simulink model "U27Estim"  (R2022b)
settings: Solver=ode23  StartTime=0.0  StopTime=2  RelTol=1e-3
undefined symbols (not defined in the file or in its folder): b, f, J, Kcj, Lm, Lr, Ls, p, Rr, Rs, Vs
libraries: cstblocks x2, spsAsynchronousMachineSIUnitsLib x1, spsGroundLib x1, spsThreePhaseProgrammableVoltageSourceLib x1, spsThreePhaseVIMeasurementLib x1, spspowerguiLib x1, spsPLL3phLib x1, spsabctodq0Lib x1
settings Model: Creator=automatizacion  LastModifiedBy=electronica

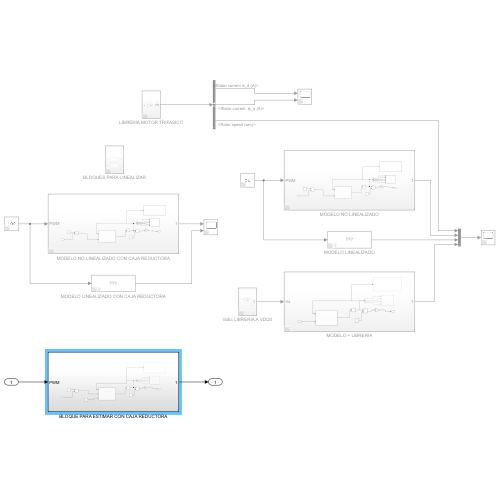
[thumbnail: Simulink's stored preview of the top-level diagram]
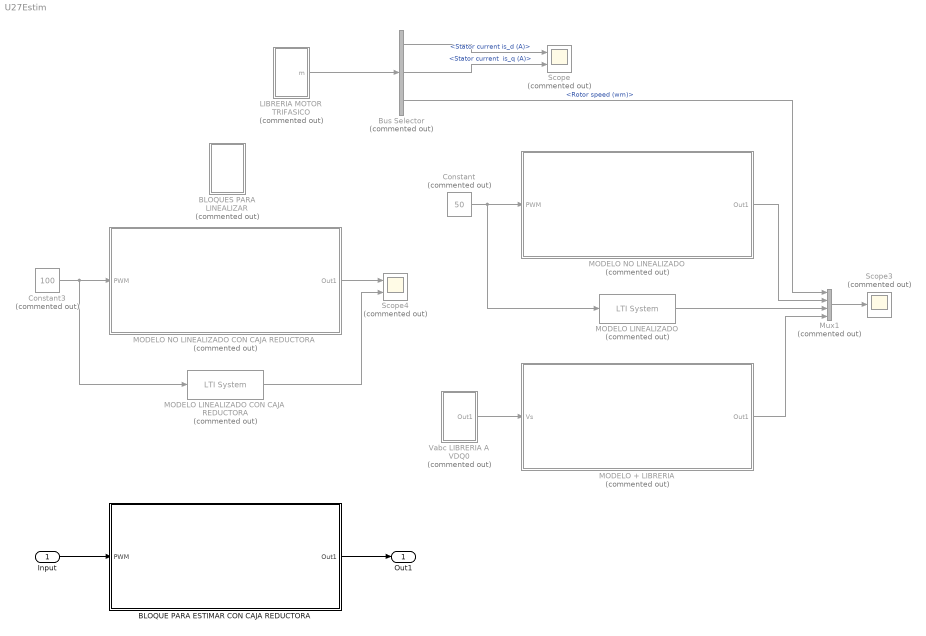
== system U27Estim ==
  Input : Inport
  BLOQUE PARA ESTIMAR CON CAJA REDUCTORA : Subsystem
  BLOQUES PARA LINEALIZAR : Subsystem  Commented=on
  Bus Selector : BusSelector  Commented=on  OutputSignals="Stator measurements.Stator current is_d (A),Stator measurements.Stator current  is_q (A),Mechanical.Rotor speed (wm)"
  Constant : Constant  Commented=on  Value=50
  Constant3 : Constant  Commented=on  Value=100
  LIBRERIA MOTOR TRIFASICO : Subsystem  Commented=on
  MODELO + LIBRERIA : Subsystem  Commented=on
  "MODELO LINEALIZADO " : cstblocks/LTI System  Commented=on  sys=G1  IC=[]
  MODELO LINEALIZADO CON CAJA REDUCTORA : cstblocks/LTI System  Commented=on  sys=G2  IC=[]
  "MODELO NO LINEALIZADO " : Subsystem  Commented=on
  MODELO NO LINEALIZADO CON CAJA REDUCTORA : Subsystem  Commented=on
  Mux1 : Mux  Commented=on
  Scope : Scope  Commented=on  NumInputPorts=2
  Scope3 : Scope  Commented=on
  Scope4 : Scope  Commented=on  NumInputPorts=2
  Vabc LIBRERIA A VDQ0 : Subsystem  Commented=on
  Out1 : Outport
  wires:
  Bus Selector/2 -> Scope/2  "<Stator current  is_q (A)>"
  Bus Selector/1 -> Scope/1  "<Stator current is_d (A)>"
  Mux1/1 -> Scope3/1
  Constant/1 -> "MODELO LINEALIZADO "/1, "MODELO NO LINEALIZADO "/1(PWM)
  Bus Selector/3 -> Mux1/1  "<Rotor speed (wm)>"
  "MODELO NO LINEALIZADO "/1(Out1) -> Mux1/2
  MODELO + LIBRERIA/1(Out1) -> Mux1/4
  "MODELO LINEALIZADO "/1 -> Mux1/3
  MODELO NO LINEALIZADO CON CAJA REDUCTORA/1(Out1) -> Scope4/1
  Constant3/1 -> MODELO LINEALIZADO CON CAJA REDUCTORA/1, MODELO NO LINEALIZADO CON CAJA REDUCTORA/1(PWM)
  MODELO LINEALIZADO CON CAJA REDUCTORA/1 -> Scope4/2
  Vabc LIBRERIA A VDQ0/1(Out1) -> MODELO + LIBRERIA/1(Vs)
  LIBRERIA MOTOR TRIFASICO/1(m) -> Bus Selector/1
  Input/1 -> BLOQUE PARA ESTIMAR CON CAJA REDUCTORA/1(PWM)
  BLOQUE PARA ESTIMAR CON CAJA REDUCTORA/1(Out1) -> Out1/1

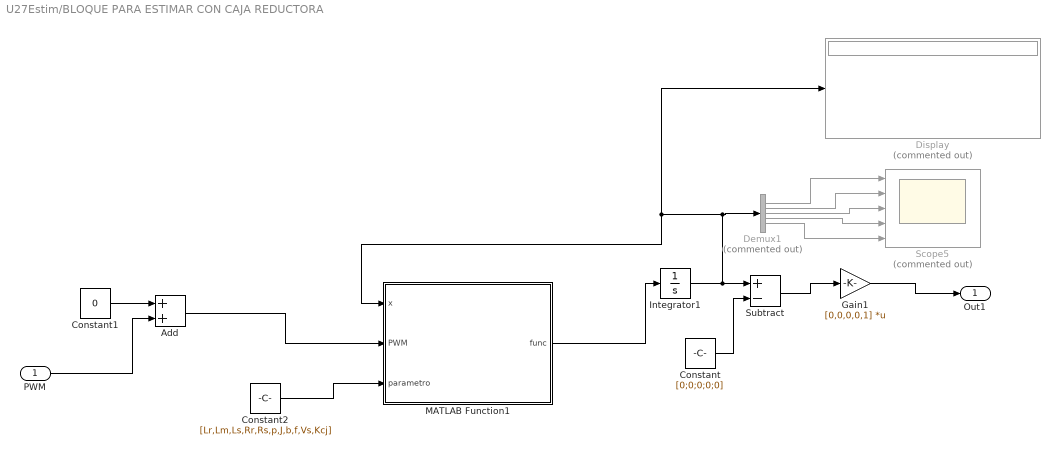
== system U27Estim/BLOQUE PARA ESTIMAR CON CAJA REDUCTORA ==
  PWM : Inport
  Add : Sum
  Constant : Constant  Value=[0;0;0;0;0]
  Constant1 : Constant  Value=0
  Constant2 : Constant  Value=[Lr,Lm,Ls,Rr,Rs,p,J,b,f,Vs,Kcj]
  Demux1 : Demux  Commented=on  Outputs=5
  Display : Display  Commented=on
  Gain1 : Gain  Gain=[0,0,0,0,1]  Multiplication=Matrix(K*u)
  Integrator1 : Integrator  InitialCondition=[0;0;0;0;0]
  MATLAB Function1 : MATLAB Function  TreatAsAtomicUnit=on
  Scope5 : Scope  Commented=on  NumInputPorts=5
  Subtract : Sum  Inputs=+-
  Out1 : Outport
  wires:
  Demux1/2 -> Scope5/2
  MATLAB Function1/1(func) -> Integrator1/1
  Integrator1/1 -> Demux1/1, Display/1, MATLAB Function1/1(x), Subtract/1
  Demux1/1 -> Scope5/1
  Demux1/4 -> Scope5/4
  Gain1/1 -> Out1/1
  Demux1/3 -> Scope5/3
  Constant/1 -> Subtract/2
  Subtract/1 -> Gain1/1
  Constant1/1 -> Add/1
  PWM/1 -> Add/2
  Add/1 -> MATLAB Function1/2(PWM)
  Demux1/5 -> Scope5/5
  Constant2/1 -> MATLAB Function1/3(parametro)

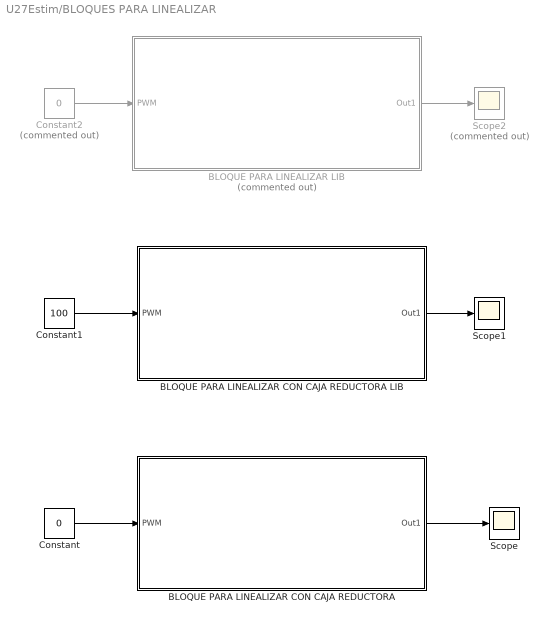
== system U27Estim/BLOQUES PARA LINEALIZAR ==
  BLOQUE PARA LINEALIZAR CON CAJA REDUCTORA : Subsystem
  BLOQUE PARA LINEALIZAR CON CAJA REDUCTORA LIB : Subsystem
  BLOQUE PARA LINEALIZAR LIB : Subsystem  Commented=on
  Constant : Constant  Value=0
  Constant1 : Constant  Value=100
  Constant2 : Constant  Commented=on  Value=0
  Scope : Scope
  Scope1 : Scope
  Scope2 : Scope  Commented=on
  wires:
  Constant2/1 -> BLOQUE PARA LINEALIZAR LIB/1(PWM)
  BLOQUE PARA LINEALIZAR LIB/1(Out1) -> Scope2/1
  Constant1/1 -> BLOQUE PARA LINEALIZAR CON CAJA REDUCTORA LIB/1(PWM)
  BLOQUE PARA LINEALIZAR CON CAJA REDUCTORA LIB/1(Out1) -> Scope1/1
  BLOQUE PARA LINEALIZAR CON CAJA REDUCTORA/1(Out1) -> Scope/1
  Constant/1 -> BLOQUE PARA LINEALIZAR CON CAJA REDUCTORA/1(PWM)

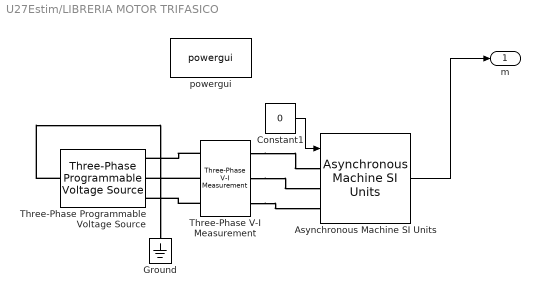
== system U27Estim/LIBRERIA MOTOR TRIFASICO ==
  Asynchronous Machine SI Units : spsAsynchronousMachineSIUnitsLib/Asynchronous Machine SI Units  RotorType=Squirrel-cage  PresetModel="01:  5 HP   460 V 60Hz 1750 RPM"  MechanicalLoad=Torque Tm  ShowDetailedParameters=on  ReferenceFrame=Synchronous  Units=SI  MeasurementBus=off  NominalParameters=[3730 460 60]  VoltageRatio=1  Stator=[1.115 0.005974]  Rotor=[1.083 0.005974]  Cage1=[0.4155 0.002066]  Cage2=[0.4168 0.0003495]  Lm=0.2037  Mechanical=[0.02 0.005752 2]  PolePairs=2  InitialConditions=[1 1 0 0 0 0 0 0]  SimulateSaturation=off  Saturation=[14.03593122, 27.81365428, 53.79336849, 72.68890987, 97.98006896, 148.6815601, 215.7428561, 302.9841135, 428.7778367 ; 230, 322, 414, 460, 506, 552, 598, 644, 690]  LoadFlowParameters=1492000  TsPowergui=0  TsBlock=-1  IterativeModel=Trapezoidal non iterative  IterativeDiscreteModel=Trapezoidal non iterative  Pmec=1.492e+006
  Constant1 : Constant  Value=0
  Ground : spsGroundLib/Ground  LConnTagsString=a
  Three-Phase Programmable Voltage Source : spsThreePhaseProgrammableVoltageSourceLib/Three-Phase Programmable Voltage Source  PositiveSequence="[460  0 30]"  VariationEntity=None  VariationType=Table of time-amplitude pairs  VariationTypeAlt=Step  VariationStep=0.5  VariationRate=10  VariationMagnitude=0.3  VariationFrequency=2  VariationTiming=[1 2]  VariationPhaseA=off  Amplitudes=[1 0.8 1.2 1.0]  TimeValues=[0 0.1 0.15 0.2]  HarmonicGeneration=off  HarmonicA=[3 0.2 -25 0]  HarmonicB=[2 0.15 35 2]  Timing="[0.05  3]"  BusType=swing  Pref=0  Qref=0  Qmin=-inf  Qmax=inf
  Three-Phase V-I Measurement : spsThreePhaseVIMeasurementLib/Three-Phase V-I Measurement  VoltageMeasurement=phase-to-ground  SetLabelV=on  LabelV=Vabc  Vpu=off  VpuLL=off  CurrentMeasurement=yes  SetLabelI=on  LabelI=Iabc  Ipu=off  Pbase=100e6  Vbase=500e3  OutputType=Complex  PhasorSimulation=off  PSBequivalent=0
  powergui : spspowerguiLib/powergui  Priority=1  SimulationMode=Continuous  SampleTime=50e-6  frequency=60  Iterations=50  frequencyindice=60  Pbase=100e6  ErrMax=1e-4  UnitsV=kV  UnitsW=MW  buscounter=0  FunctionMessages=off  echomessages=off  EnableUseOfTLC=off  CurrentSourceSwitches=off  DisableSnubberDevices=off  DisableRonSwitches=off  DisableVfSwitches=off  DisplayEquations=off  AutomaticDiscreteSolvers=off  SolverType=Tustin/Backward Euler (TBE)  Interpol=off  ExternalGateDelay=off  methode=off  Ts=100  x0status=blocks  SPID=on  SwTol=0  HookPort=off  NonlinearTolerance=1e-4  nMaxIteration=100  ContinueOnMaxIteration=off  RestoreLinks=warning  ResistiveCurrentMeasurement=off  Frange=[0:2:500]  Ylog=off  Xlog=on  ShowGrid=off  save=off  variable=ZData  structure=0  ZoomFFT=off  StartTime=0.0  cycles=1  DisplayStyle=1  fundamental=60  FreqAxis=off  MaxFrequency=1000  frequencyindicesteady=1  RmsSteady=1  display=off
  m : Outport
  wires:
  Asynchronous Machine SI Units/1 -> m/1
  Constant1/1 -> Asynchronous Machine SI Units/1
  connections:
  Three-Phase V-I Measurement/RConn1 -- Asynchronous Machine SI Units/LConn1
  Three-Phase V-I Measurement/LConn3 -- Three-Phase Programmable Voltage Source/RConn3
  Three-Phase V-I Measurement/LConn1 -- Three-Phase Programmable Voltage Source/RConn1
  Three-Phase Programmable Voltage Source/LConn1 -- Ground/LConn1
  Three-Phase V-I Measurement/RConn2 -- Asynchronous Machine SI Units/LConn2
  Three-Phase V-I Measurement/RConn3 -- Asynchronous Machine SI Units/LConn3
  Three-Phase V-I Measurement/LConn2 -- Three-Phase Programmable Voltage Source/RConn2

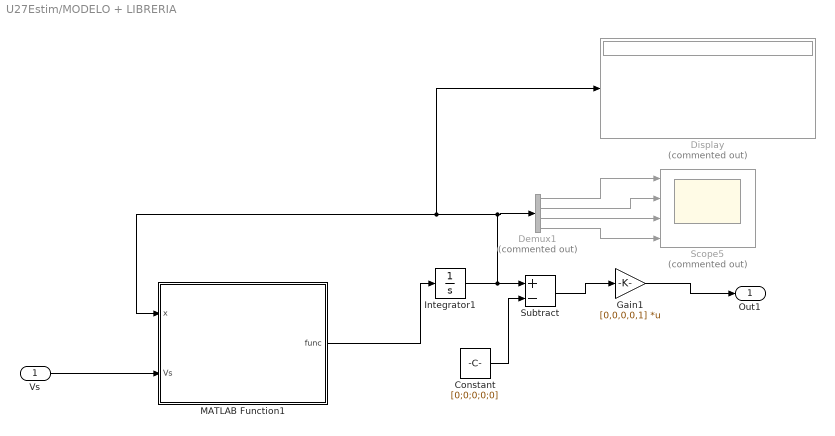
== system U27Estim/MODELO + LIBRERIA ==
  Vs : Inport
  Constant : Constant  Value=[0;0;0;0;0]
  Demux1 : Demux  Commented=on
  Display : Display  Commented=on
  Gain1 : Gain  Gain=[0,0,0,0,1]  Multiplication=Matrix(K*u)
  Integrator1 : Integrator  InitialCondition=[0;0;0;0;0]
  MATLAB Function1 : MATLAB Function  TreatAsAtomicUnit=on
  Scope5 : Scope  Commented=on  NumInputPorts=4
  Subtract : Sum  Inputs=+-
  Out1 : Outport
  wires:
  Demux1/2 -> Scope5/2
  MATLAB Function1/1(func) -> Integrator1/1
  Integrator1/1 -> Demux1/1, Display/1, MATLAB Function1/1(x), Subtract/1
  Demux1/1 -> Scope5/1
  Demux1/4 -> Scope5/4
  Gain1/1 -> Out1/1
  Demux1/3 -> Scope5/3
  Constant/1 -> Subtract/2
  Subtract/1 -> Gain1/1
  Vs/1 -> MATLAB Function1/2(Vs)

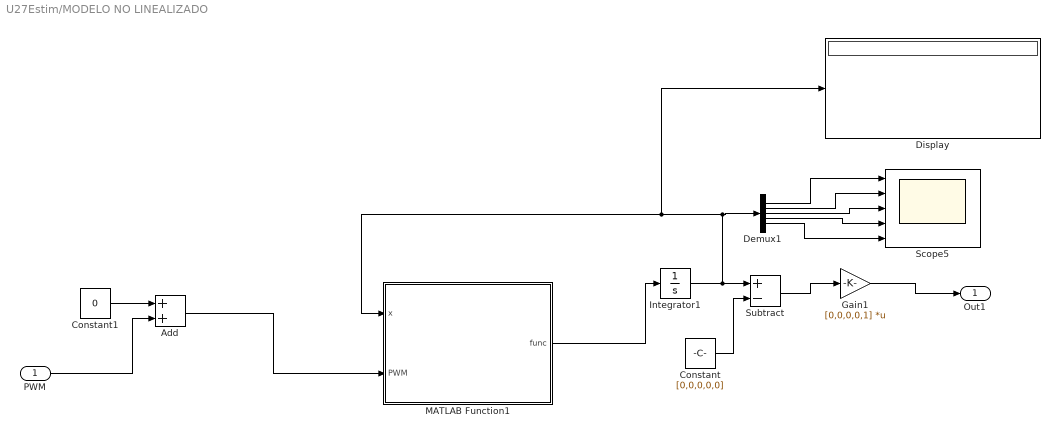
== system U27Estim/MODELO NO LINEALIZADO  ==
  PWM : Inport
  Add : Sum
  Constant : Constant  Value=[0,0,0,0,0]
  Constant1 : Constant  Value=0
  Demux1 : Demux  Outputs=5
  Display : Display
  Gain1 : Gain  Gain=[0,0,0,0,1]  Multiplication=Matrix(K*u)
  Integrator1 : Integrator  InitialCondition=[0,0,0,0,0]
  MATLAB Function1 : MATLAB Function  TreatAsAtomicUnit=on
  Scope5 : Scope  NumInputPorts=5
  Subtract : Sum  Inputs=+-
  Out1 : Outport
  wires:
  Demux1/2 -> Scope5/2
  MATLAB Function1/1(func) -> Integrator1/1
  Integrator1/1 -> Demux1/1, Display/1, MATLAB Function1/1(x), Subtract/1
  Demux1/1 -> Scope5/1
  Demux1/4 -> Scope5/4
  Gain1/1 -> Out1/1
  Demux1/3 -> Scope5/3
  Constant/1 -> Subtract/2
  Subtract/1 -> Gain1/1
  Constant1/1 -> Add/1
  PWM/1 -> Add/2
  Add/1 -> MATLAB Function1/2(PWM)
  Demux1/5 -> Scope5/5

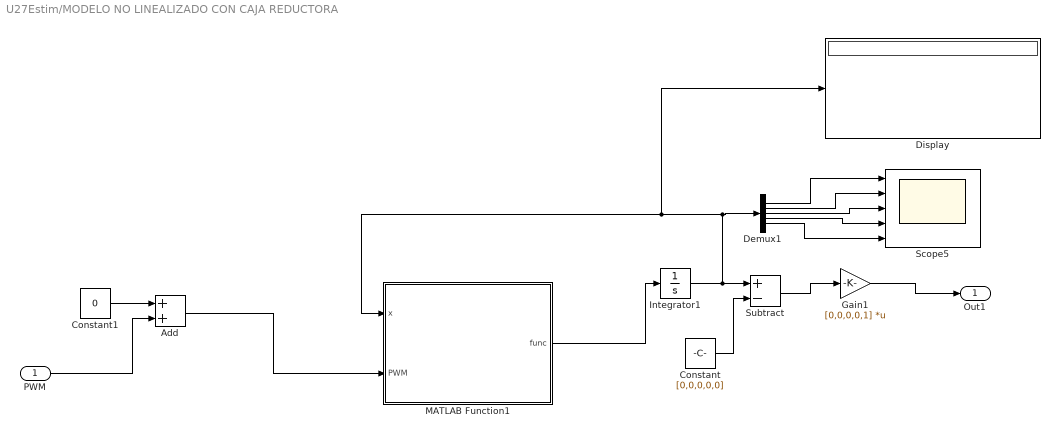
== system U27Estim/MODELO NO LINEALIZADO CON CAJA REDUCTORA ==
  PWM : Inport
  Add : Sum
  Constant : Constant  Value=[0,0,0,0,0]
  Constant1 : Constant  Value=0
  Demux1 : Demux  Outputs=5
  Display : Display
  Gain1 : Gain  Gain=[0,0,0,0,1]  Multiplication=Matrix(K*u)
  Integrator1 : Integrator  InitialCondition=[0,0,0,0,0]
  MATLAB Function1 : MATLAB Function  TreatAsAtomicUnit=on
  Scope5 : Scope  NumInputPorts=5
  Subtract : Sum  Inputs=+-
  Out1 : Outport
  wires:
  Demux1/2 -> Scope5/2
  MATLAB Function1/1(func) -> Integrator1/1
  Integrator1/1 -> Demux1/1, Display/1, MATLAB Function1/1(x), Subtract/1
  Demux1/1 -> Scope5/1
  Demux1/4 -> Scope5/4
  Gain1/1 -> Out1/1
  Demux1/3 -> Scope5/3
  Constant/1 -> Subtract/2
  Subtract/1 -> Gain1/1
  Constant1/1 -> Add/1
  PWM/1 -> Add/2
  Add/1 -> MATLAB Function1/2(PWM)
  Demux1/5 -> Scope5/5

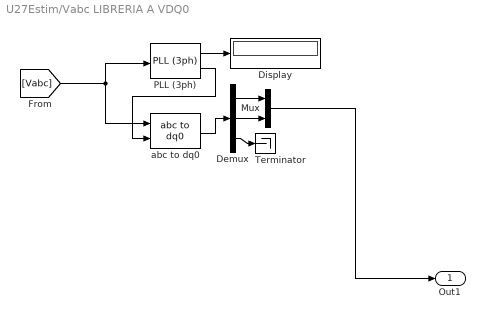
== system U27Estim/Vabc LIBRERIA A VDQ0 ==
  Demux : Demux  Outputs=3
  Display : Display
  Mux : Mux  Inputs=2
  PLL (3ph) : spsPLL3phLib/PLL (3ph)  Fmin=45  Par_Init=[0, 60]  ParK=[180, 3200, 1]  TcD=1e-4  MaxRateChangeFreq=12  FilterCutOffFreq=25  Ts=0  AGC=on
  Terminator : Terminator
  abc to dq0 : spsabctodq0Lib/abc to dq0  Alignment=90 degrees behind phase A axis
  Out1 : Outport
  wires:
  PLL (3ph)/2 -> abc to dq0/2
  [Vabc] -> abc to dq0/1, PLL (3ph)/1
  PLL (3ph)/1 -> Display/1
  Demux/3 -> Terminator/1
  Mux/1 -> Out1/1
  abc to dq0/1 -> Demux/1
  Demux/1 -> Mux/1
  Demux/2 -> Mux/2

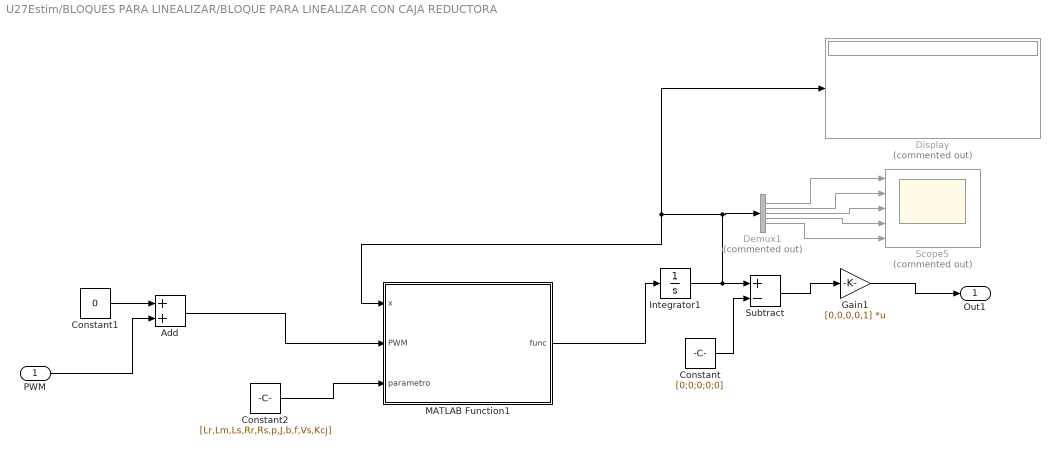
== system U27Estim/BLOQUES PARA LINEALIZAR/BLOQUE PARA LINEALIZAR CON CAJA REDUCTORA ==
  PWM : Inport
  Add : Sum
  Constant : Constant  Value=[0;0;0;0;0]
  Constant1 : Constant  Value=0
  Constant2 : Constant  Value=[Lr,Lm,Ls,Rr,Rs,p,J,b,f,Vs,Kcj]
  Demux1 : Demux  Commented=on  Outputs=5
  Display : Display  Commented=on
  Gain1 : Gain  Gain=[0,0,0,0,1]  Multiplication=Matrix(K*u)
  Integrator1 : Integrator  InitialCondition=[0;0;0;0;0]
  MATLAB Function1 : MATLAB Function  TreatAsAtomicUnit=on
  Scope5 : Scope  Commented=on  NumInputPorts=5
  Subtract : Sum  Inputs=+-
  Out1 : Outport
  wires:
  Demux1/2 -> Scope5/2
  MATLAB Function1/1(func) -> Integrator1/1
  Integrator1/1 -> Demux1/1, Display/1, MATLAB Function1/1(x), Subtract/1
  Demux1/1 -> Scope5/1
  Demux1/4 -> Scope5/4
  Gain1/1 -> Out1/1
  Demux1/3 -> Scope5/3
  Constant/1 -> Subtract/2
  Subtract/1 -> Gain1/1
  Constant1/1 -> Add/1
  PWM/1 -> Add/2
  Add/1 -> MATLAB Function1/2(PWM)
  Demux1/5 -> Scope5/5
  Constant2/1 -> MATLAB Function1/3(parametro)

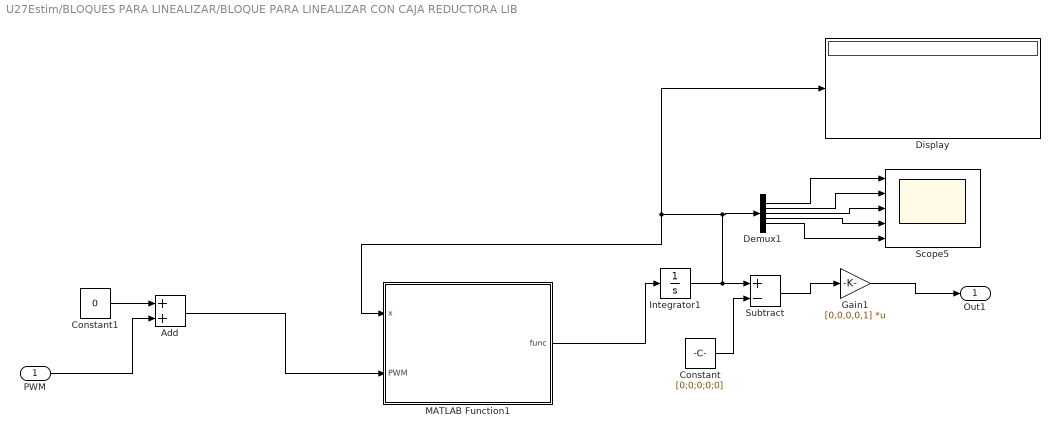
== system U27Estim/BLOQUES PARA LINEALIZAR/BLOQUE PARA LINEALIZAR CON CAJA REDUCTORA LIB ==
  PWM : Inport
  Add : Sum
  Constant : Constant  Value=[0;0;0;0;0]
  Constant1 : Constant  Value=0
  Demux1 : Demux  Outputs=5
  Display : Display
  Gain1 : Gain  Gain=[0,0,0,0,1]  Multiplication=Matrix(K*u)
  Integrator1 : Integrator  InitialCondition=[0;0;0;0;0]
  MATLAB Function1 : MATLAB Function  TreatAsAtomicUnit=on
  Scope5 : Scope  NumInputPorts=5
  Subtract : Sum  Inputs=+-
  Out1 : Outport
  wires:
  Demux1/2 -> Scope5/2
  MATLAB Function1/1(func) -> Integrator1/1
  Integrator1/1 -> Demux1/1, Display/1, MATLAB Function1/1(x), Subtract/1
  Demux1/1 -> Scope5/1
  Demux1/4 -> Scope5/4
  Gain1/1 -> Out1/1
  Demux1/3 -> Scope5/3
  Constant/1 -> Subtract/2
  Subtract/1 -> Gain1/1
  Constant1/1 -> Add/1
  PWM/1 -> Add/2
  Add/1 -> MATLAB Function1/2(PWM)
  Demux1/5 -> Scope5/5

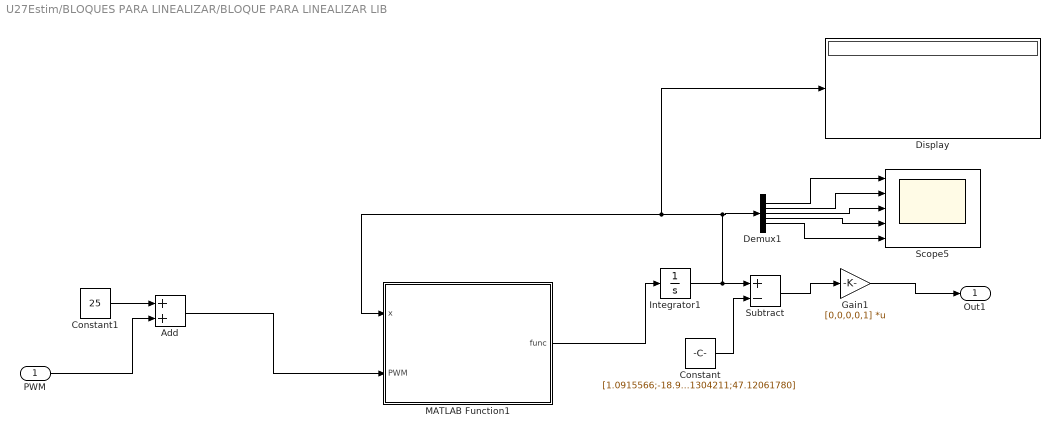
== system U27Estim/BLOQUES PARA LINEALIZAR/BLOQUE PARA LINEALIZAR LIB ==
  PWM : Inport
  Add : Sum
  Constant : Constant  Value=[1.0915566;-18.9439806;-0.02333667;-0.001304211;47.12061780]
  Constant1 : Constant  Value=25
  Demux1 : Demux  Outputs=5
  Display : Display
  Gain1 : Gain  Gain=[0,0,0,0,1]  Multiplication=Matrix(K*u)
  Integrator1 : Integrator  InitialCondition=[1.0915566;-18.9439806;-0.02333667;-0.001304211;47.12061780]
  MATLAB Function1 : MATLAB Function  TreatAsAtomicUnit=on
  Scope5 : Scope  NumInputPorts=5
  Subtract : Sum  Inputs=+-
  Out1 : Outport
  wires:
  Demux1/2 -> Scope5/2
  MATLAB Function1/1(func) -> Integrator1/1
  Integrator1/1 -> Demux1/1, Display/1, MATLAB Function1/1(x), Subtract/1
  Demux1/1 -> Scope5/1
  Demux1/4 -> Scope5/4
  Gain1/1 -> Out1/1
  Demux1/3 -> Scope5/3
  Constant/1 -> Subtract/2
  Subtract/1 -> Gain1/1
  Constant1/1 -> Add/1
  PWM/1 -> Add/2
  Add/1 -> MATLAB Function1/2(PWM)
  Demux1/5 -> Scope5/5

== matlab function U27Estim/MODELO NO LINEALIZADO /MATLAB Function1 ==
  data: x input; PWM input; func output
function func = fcn(x,PWM)
%Parametros
% Lr = parametro(1);
% Lm = parametro(2);
% Ls = parametro(3);
% Rr = parametro(4);
% Rs = parametro(5);
% p = parametro(6);
% J = parametro(7);
% b = parametro(8);
% f = parametro(9);
% Kcj = parametro(10);

Lr = 0.005974;%1
Lm = 0.2037;%2
Ls = 0.005974;%3
Rr = 1.083;%4
Rs = 1.115;%5
p = 2;%6
J = 0.02;%7
b = 0.005752;%8
f = 60;%7
Vs = 375.6;
Kcj = 1/40;

%Estados
Ids = x(1);
Iqs = x(2);
Idr = x(3);
Iqr = x(4);
wm = x(5);

% Vds = Vs(1);
% Vqs = Vs(2);

delta = (Lr+Lm)*(Ls+Lm)-Lm^2;
ws = 2*pi*(f*PWM/100);
% ws = 2*pi*(f);

R = [Rs 0 0 0;
      0 Rs 0 0;
      0 0 Rr 0;
      0 0 0 Rr];

omega = [0, -ws, 0, 0;
    ws, 0, 0, 0;
    0, 0, 0, -(ws-(p*wm));
    0, 0, (ws-(p*wm)), 0];

L = [Ls+Lm, 0, Lm, 0;
    0, Ls+Lm 0, Lm;
    Lm, 0, Lr+Lm, 0;
    0, Lm, 0, Lr+Lm];

% inv_L = (1/delta)*[Lr+Lm, 0, -Lm, 0;
%                   0, Lr+Lm, 0, -Lm;
%                   -Lm, 0, Ls+Lm, 0;
%                   0, -Lm, 0, Ls+Lm];

% Vqs = 4.889*(f*PWM/100)+16.15;

% Vs = 6.25*(f*PWM/100);


% V = [Vds;
%        Vqs;
%        0;
%        0];
   
   V = [Vs;
       0;
       0;
       0];


I = [Ids;
    Iqs;
    Idr;
    Iqr];

dI = -(inv(L)*R + inv(L)*omega*L)*I + inv(L)*V;
Te = 1.5*p*Lm*(Iqs*Idr - Ids*Iqr);
dwm = (1/J)*(Te - (b)*wm);
func = [dI; dwm];

== matlab function U27Estim/MODELO + LIBRERIA/MATLAB Function1 ==
  data: x input; Vs input; func output
function func = fcn(x,Vs)
%Parametros
% Lr = parametro(1);
% Lm = parametro(2);
% Ls = parametro(3);
% Rr = parametro(4);
% Rs = parametro(5);
% p = parametro(6);
% J = parametro(7);
% b = parametro(8);
% f = parametro(9);
% Kcj = parametro(10);

Lr = 0.005974;%1
Lm = 0.2037;%2
Ls = 0.005974;%3
Rr = 1.083;%4
Rs = 1.115;%5
p = 2;%6
J = 0.02;%7
b = 0.005752;%8
f = 60;%7
% Vs = 460;
Kcj = 1/40;

%Estados
Ids = x(1);
Iqs = x(2);
Idr = x(3);
Iqr = x(4);
wm = x(5);

Vds = Vs(1);
Vqs = Vs(2);

delta = (Lr+Lm)*(Ls+Lm)-Lm^2;
ws = 2*pi*f;
% ws = 2*pi*(f);

R = [Rs 0 0 0;
      0 Rs 0 0;
      0 0 Rr 0;
      0 0 0 Rr];

omega = [0, -ws, 0, 0;
    ws, 0, 0, 0;
    0, 0, 0, -(ws-(p*wm));
    0, 0, (ws-(p*wm)), 0];

L = [Ls+Lm, 0, Lm, 0;
    0, Ls+Lm 0, Lm;
    Lm, 0, Lr+Lm, 0;
    0, Lm, 0, Lr+Lm];

% inv_L = (1/delta)*[Lr+Lm, 0, -Lm, 0;
%                   0, Lr+Lm, 0, -Lm;
%                   -Lm, 0, Ls+Lm, 0;
%                   0, -Lm, 0, Ls+Lm];

% Vqs = 4.889*(f*PWM/100)+16.15;

% Vs = 6.25*(f*PWM/100);


% V = [Vds;
%        Vqs;
%        0;
%        0];
   
   V = [Vds;
       Vqs;
       0;
       0];


I = [Ids;
    Iqs;
    Idr;
    Iqr];

dI = -(inv(L)*R + inv(L)*omega*L)*I + inv(L)*V;
Te = 1.5*p*Lm*(Iqs*Idr - Ids*Iqr);
dwm = (1/J)*(Te - (b)*wm);
func = [dI; dwm];

== matlab function U27Estim/BLOQUES PARA LINEALIZAR/BLOQUE PARA LINEALIZAR LIB/MATLAB Function1 ==
  data: x input; PWM input; func output
function func = fcn(x,PWM)
%Parametros
% Lr = parametro(1);
% Lm = parametro(2);
% Ls = parametro(3);
% Rr = parametro(4);
% Rs = parametro(5);
% p = parametro(6);
% J = parametro(7);
% b = parametro(8);
% f = parametro(9);
% Kcj = parametro(10);

Lr = 0.005974;%1
Lm = 0.2037;%2
Ls = 0.005974;%3
Rr = 1.083;%4
Rs = 1.115;%5
p = 2;%6
J = 0.02;%7
b = 0.005752;%8
f = 60;%7
Vs = 375.6;
Kcj = 1/40;

%Estados
Ids = x(1);
Iqs = x(2);
Idr = x(3);
Iqr = x(4);
wm = x(5);

% Vds = Vs(1);
% Vqs = Vs(2);

delta = (Lr+Lm)*(Ls+Lm)-Lm^2;
ws = 2*pi*(f*PWM/100);
% ws = 2*pi*(f);

R = [Rs 0 0 0;
      0 Rs 0 0;
      0 0 Rr 0;
      0 0 0 Rr];

omega = [0, -ws, 0, 0;
    ws, 0, 0, 0;
    0, 0, 0, -(ws-(p*wm));
    0, 0, (ws-(p*wm)), 0];

L = [Ls+Lm, 0, Lm, 0;
    0, Ls+Lm 0, Lm;
    Lm, 0, Lr+Lm, 0;
    0, Lm, 0, Lr+Lm];

% inv_L = (1/delta)*[Lr+Lm, 0, -Lm, 0;
%                   0, Lr+Lm, 0, -Lm;
%                   -Lm, 0, Ls+Lm, 0;
%                   0, -Lm, 0, Ls+Lm];

% Vqs = 4.889*(f*PWM/100)+16.15;

% Vs = 6.25*(f*PWM/100);


% V = [Vds;
%        Vqs;
%        0;
%        0];
   
   V = [Vs;
       0;
       0;
       0];


I = [Ids;
    Iqs;
    Idr;
    Iqr];

dI = -(inv(L)*R + inv(L)*omega*L)*I + inv(L)*V;
Te = 1.5*p*Lm*(Iqs*Idr - Ids*Iqr);
dwm = (1/J)*(Te - (b)*wm);
func = [dI; dwm];

== matlab function U27Estim/MODELO NO LINEALIZADO CON CAJA REDUCTORA/MATLAB Function1 ==
  data: x input; PWM input; func output
function func = fcn(x,PWM)
%Parametros
% Lr = parametro(1);
% Lm = parametro(2);
% Ls = parametro(3);
% Rr = parametro(4);
% Rs = parametro(5);
% p = parametro(6);
% J = parametro(7);
% b = parametro(8);
% f = parametro(9);
% Kcj = parametro(10);

Lr = 0.005974;%1
Lm = 0.2037;%2
Ls = 0.005974;%3
Rr = 1.083;%4
Rs = 1.115;%5
p = 2;%6
J = 0.02;%7
b = 0.005752;%8
f = 60;%7
Vs = 375.6;
Kcj = 1/40;

%Estados
Ids = x(1);
Iqs = x(2);
Idr = x(3);
Iqr = x(4);
wm = x(5);

% Vds = Vs(1);
% Vqs = Vs(2);

delta = (Lr+Lm)*(Ls+Lm)-Lm^2;
ws = 2*pi*(f*PWM/100)*Kcj;
% ws = 2*pi*(f);

R = [Rs 0 0 0;
      0 Rs 0 0;
      0 0 Rr 0;
      0 0 0 Rr];

omega = [0, -ws, 0, 0;
    ws, 0, 0, 0;
    0, 0, 0, -(ws-(p*wm));
    0, 0, (ws-(p*wm)), 0];

L = [Ls+Lm, 0, Lm, 0;
    0, Ls+Lm 0, Lm;
    Lm, 0, Lr+Lm, 0;
    0, Lm, 0, Lr+Lm];

% inv_L = (1/delta)*[Lr+Lm, 0, -Lm, 0;
%                   0, Lr+Lm, 0, -Lm;
%                   -Lm, 0, Ls+Lm, 0;
%                   0, -Lm, 0, Ls+Lm];

% Vqs = 4.889*(f*PWM/100)+16.15;

% Vs = 6.25*(f*PWM/100);


% V = [Vds;
%        Vqs;
%        0;
%        0];
   
   V = [Vs;
       0;
       0;
       0];


I = [Ids;
    Iqs;
    Idr;
    Iqr];

dI = -(inv(L)*R + inv(L)*omega*L)*I + inv(L)*V;
Te = 1.5*p*Lm*(Iqs*Idr - Ids*Iqr);
dwm = (1/J)*(Te*Kcj - (b)*wm);
func = [dI; dwm*Kcj];

== matlab function U27Estim/BLOQUES PARA LINEALIZAR/BLOQUE PARA LINEALIZAR CON CAJA REDUCTORA LIB/MATLAB Function1 ==
  data: x input; PWM input; func output
function func = fcn(x,PWM)
%Parametros
% Lr = parametro(1);
% Lm = parametro(2);
% Ls = parametro(3);
% Rr = parametro(4);
% Rs = parametro(5);
% p = parametro(6);
% J = parametro(7);
% b = parametro(8);
% f = parametro(9);
% Vs = parametro(10);
% Kcj = parametro(11);

Lr = 0.005974;%1
Lm = 0.2037;%2
Ls = 0.005974;%3
Rr = 1.083;%4
Rs = 1.115;%5
p = 2;%6
J = 0.02;%7
b = 0.005752;%8
f = 60;%7
Vs = 375.6;
Kcj = 1/40;

%Estados
Ids = x(1);
Iqs = x(2);
Idr = x(3);
Iqr = x(4);
wm = x(5);

% Vds = Vs(1);
% Vqs = Vs(2);

delta = (Lr+Lm)*(Ls+Lm)-Lm^2;
ws = 2*pi*(f*PWM/100)*Kcj;
% ws = 2*pi*(f);

R = [Rs 0 0 0;
      0 Rs 0 0;
      0 0 Rr 0;
      0 0 0 Rr];

omega = [0, -ws, 0, 0;
    ws, 0, 0, 0;
    0, 0, 0, -(ws-(p*wm));
    0, 0, (ws-(p*wm)), 0];

L = [Ls+Lm, 0, Lm, 0;
    0, Ls+Lm 0, Lm;
    Lm, 0, Lr+Lm, 0;
    0, Lm, 0, Lr+Lm];

% inv_L = (1/delta)*[Lr+Lm, 0, -Lm, 0;
%                   0, Lr+Lm, 0, -Lm;
%                   -Lm, 0, Ls+Lm, 0;
%                   0, -Lm, 0, Ls+Lm];

% Vqs = 4.889*(f*PWM/100)+16.15;

% Vs = 6.25*(f*PWM/100);


% V = [Vds;
%        Vqs;
%        0;
%        0];
   
   V = [Vs;
       0;
       0;
       0];


I = [Ids;
    Iqs;
    Idr;
    Iqr];

dI = -(inv(L)*R + inv(L)*omega*L)*I + inv(L)*V;
Te = 1.5*p*Lm*(Iqs*Idr - Ids*Iqr);
dwm = (1/J)*Kcj*(Te - (b)*wm);
func = [dI; dwm];

== matlab function U27Estim/BLOQUE PARA ESTIMAR CON CAJA REDUCTORA/MATLAB Function1 ==
  data: x input; PWM input; func output; parametro input
function func = fcn(x,PWM,parametro)
%Parametros
Lr = parametro(1);
Lm = parametro(2);
Ls = parametro(3);
Rr = parametro(4);
Rs = parametro(5);
p = parametro(6);
J = parametro(7);
b = parametro(8);
f = parametro(9);
Vs = parametro(10);
Kcj = parametro(11);

% Lr = 0.005974;%1
% Lm = 0.2037;%2
% Ls = 0.005974;%3
% Rr = 1.083;%4
% Rs = 1.115;%5
% p = 2;%6
% J = 0.02;%7
% b = 0.005752;%8
% f = 60;%7
% Vs = 375.6;
% Kcj = 1/40;

%Estados
Ids = x(1);
Iqs = x(2);
Idr = x(3);
Iqr = x(4);
wm = x(5);

% Vds = Vs(1);
% Vqs = Vs(2);

delta = (Lr+Lm)*(Ls+Lm)-Lm^2;
ws = 2*pi*(f*PWM/100)*Kcj;
% ws = 2*pi*(f);

R = [Rs 0 0 0;
      0 Rs 0 0;
      0 0 Rr 0;
      0 0 0 Rr];

omega = [0, -ws, 0, 0;
    ws, 0, 0, 0;
    0, 0, 0, -(ws-(p*wm));
    0, 0, (ws-(p*wm)), 0];

L = [Ls+Lm, 0, Lm, 0;
    0, Ls+Lm 0, Lm;
    Lm, 0, Lr+Lm, 0;
    0, Lm, 0, Lr+Lm];

% inv_L = (1/delta)*[Lr+Lm, 0, -Lm, 0;
%                   0, Lr+Lm, 0, -Lm;
%                   -Lm, 0, Ls+Lm, 0;
%                   0, -Lm, 0, Ls+Lm];

% Vqs = 4.889*(f*PWM/100)+16.15;

% Vs = 6.25*(f*PWM/100);


% V = [Vds;
%        Vqs;
%        0;
%        0];
   
   V = [Vs;
       0;
       0;
       0];


I = [Ids;
    Iqs;
    Idr;
    Iqr];

dI = -(inv(L)*R + inv(L)*omega*L)*I + inv(L)*V;
Te = 1.5*p*Lm*(Iqs*Idr - Ids*Iqr);
dwm = (1/J)*Kcj*(Te*Kcj - (b)*wm);
func = [dI; dwm];

== matlab function U27Estim/BLOQUES PARA LINEALIZAR/BLOQUE PARA LINEALIZAR CON CAJA REDUCTORA/MATLAB Function1 ==
  data: x input; PWM input; func output; parametro input
function func = fcn(x,PWM,parametro)
%Parametros
Lr = parametro(1);
Lm = parametro(2);
Ls = parametro(3);
Rr = parametro(4);
Rs = parametro(5);
p = parametro(6);
J = parametro(7);
b = parametro(8);
f = parametro(9);
Vs = parametro(10);
Kcj = parametro(11);

% Lr = 0.005974;%1
% Lm = 0.2037;%2
% Ls = 0.005974;%3
% Rr = 1.083;%4
% Rs = 1.115;%5
% p = 2;%6
% J = 0.02;%7
% b = 0.005752;%8
% f = 60;%7
% Vs = 375.6;
% Kcj = 1/40;

%Estados
Ids = x(1);
Iqs = x(2);
Idr = x(3);
Iqr = x(4);
wm = x(5);

% Vds = Vs(1);
% Vqs = Vs(2);

delta = (Lr+Lm)*(Ls+Lm)-Lm^2;
ws = 2*pi*(f*PWM/100)*Kcj;
% ws = 2*pi*(f);

R = [Rs 0 0 0;
      0 Rs 0 0;
      0 0 Rr 0;
      0 0 0 Rr];

omega = [0, -ws, 0, 0;
    ws, 0, 0, 0;
    0, 0, 0, -(ws-(p*wm));
    0, 0, (ws-(p*wm)), 0];

L = [Ls+Lm, 0, Lm, 0;
    0, Ls+Lm 0, Lm;
    Lm, 0, Lr+Lm, 0;
    0, Lm, 0, Lr+Lm];

% inv_L = (1/delta)*[Lr+Lm, 0, -Lm, 0;
%                   0, Lr+Lm, 0, -Lm;
%                   -Lm, 0, Ls+Lm, 0;
%                   0, -Lm, 0, Ls+Lm];

% Vqs = 4.889*(f*PWM/100)+16.15;

% Vs = 6.25*(f*PWM/100);


% V = [Vds;
%        Vqs;
%        0;
%        0];
   
   V = [Vs;
       0;
       0;
       0];


I = [Ids;
    Iqs;
    Idr;
    Iqr];

dI = -(inv(L)*R + inv(L)*omega*L)*I + inv(L)*V;
Te = 1.5*p*Lm*(Iqs*Idr - Ids*Iqr);
dwm = (1/J)*Kcj*(Te*Kcj - (b)*wm);
func = [dI; dwm];
